simulink library "aeroLibrary"  (R2020b)
settings: Solver=VariableStepAuto  StartTime=0.0  StopTime=10.0  RelTol=1e-3
undefined symbols (not defined in the file): aero
settings Model: Creator=ericb  LastModifiedBy=ericb

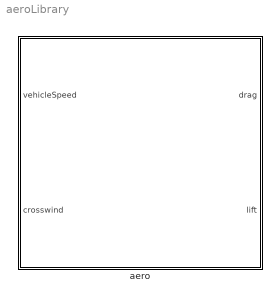
== system aeroLibrary ==
  aero : Subsystem  Variant=on

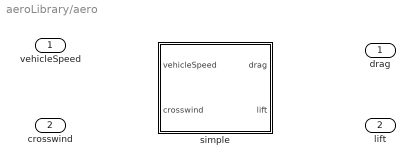
== system aeroLibrary/aero ==
  vehicleSpeed : Inport
  crosswind : Inport  Port=2
  simple : Subsystem  VariantControl=strcmp(aero.blockChoice, 'simple')
  drag : Outport
  lift : Outport  Port=2

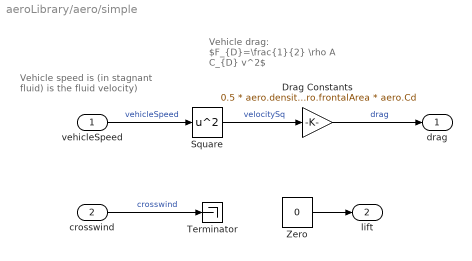
== system aeroLibrary/aero/simple ==
  note: Vehicle drag:
      | $F_{D}=\frac{1}{2} \rho A C_{D} v^2$
  note: Vehicle speed is (in stagnant fluid) is the fluid velocity)
  vehicleSpeed : Inport
  crosswind : Inport  Port=2
  Drag Constants : Gain  Gain=0.5 * aero.density * aero.frontalArea * aero.Cd
  Square : Math  Operator=square  SaturateOnIntegerOverflow=on
  Terminator : Terminator
  Zero : Constant  Value=0  OutDataTypeStr=Inherit: Inherit via back propagation
  drag : Outport
  lift : Outport  Port=2
  wires:
  crosswind/1 -> Terminator/1  "crosswind"
  Zero/1 -> lift/1
  vehicleSpeed/1 -> Square/1  "vehicleSpeed"
  Square/1 -> Drag Constants/1  "velocitySq"
  Drag Constants/1 -> drag/1  "drag"
